simulink model "lab1_2"  (R2019b)
settings: Solver=VariableStepAuto  StartTime=0.0  StopTime=100.0  RelTol=1e-3  AbsTol=10e-10
values from neighbouring files (symbols this model uses):
  den1 = cell2mat(den1)    [lab1.m]
  num1 = cell2mat(num1)    [lab1.m]
settings Model: Creator=spencersun  LastModifiedBy=spencersun

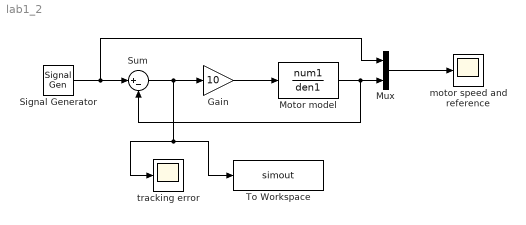
== system lab1_2 ==
  " Motor model " : TransferFcn  Numerator=num1  Denominator=den1
  Gain : Gain  Gain=10
  Mux : Mux  Inputs=2
  Signal Generator : SignalGenerator  WaveForm=square  Frequency=0.02
  Sum : Sum  Inputs=|+-
  To Workspace : ToWorkspace  VariableName=simout  SaveFormat=Timeseries  SampleTime=-1
  motor speed and reference : Scope
  "tracking error " : Scope
  wires:
  Signal Generator/1 -> Mux/1, Sum/1
  Gain/1 -> " Motor model "/1
  " Motor model "/1 -> Sum/2, Mux/2
  Sum/1 -> To Workspace/1, "tracking error "/1, Gain/1
  Mux/1 -> motor speed and reference/1
